simulink model "topology_2"  (R2024b)
settings: Solver=VariableStepAuto  StartTime=0.0  StopTime=1  RelTol=1e-3
undefined symbols (not defined in the file): C, L, par
libraries: spsSeriesRLCBranchLib x4, spsCurrentMeasurementLib x2, spsMosfetLib x2, spsVoltageMeasurementLib x2, spsDCVoltageSourceLib x1, spspowerguiLib x1
settings Model: Creator=marco  LastModifiedBy=marco

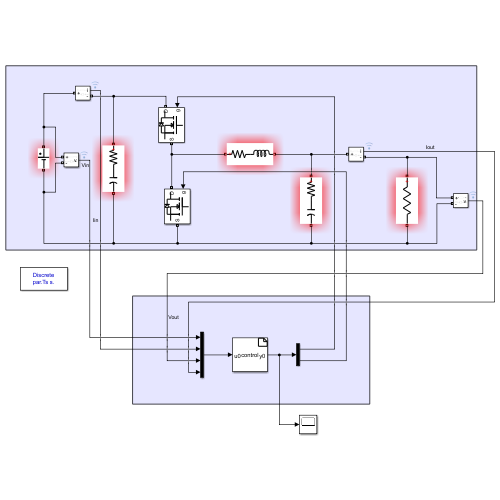
[thumbnail: Simulink's stored preview of the top-level diagram]
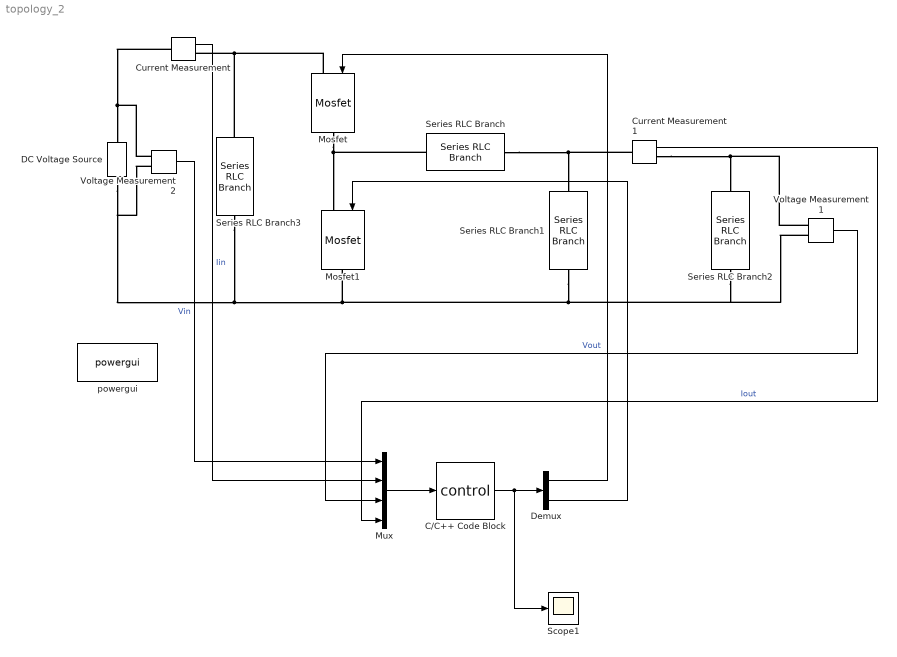
== system topology_2 ==
  C/C++ Code Block : S-Function  FunctionName=control  SFunctionModules=control_wrapper.c  SFunctionDeploymentMode=off  EnableBusSupport=off  mask(S-Function Builder){}
      mask help: Simulink:masks:SFunctionBuilder_MD
      mask init:
      | val = [[.9  0.75 0.75 1 1 .9 .9 1]',[1 1 0.75 0.75 .9 .9 1 .9]'];try , sys = get_param(gcb,'SfunBuilderFcnName');if isempty(sys), sys = get_param(gcb,'FunctionName'); end,catch, sys = get_param(gcb,'FunctionName'); end
      settings: CopyFcn=set_param(gcbh,'LinkStatus','none')  OpenFcn=sfunctionwizard(gcbh)
      mask Display:
      | plot(val(:,1),val(:,2))
      | disp(sys)
      | port_label('input',1,sprintf('%s', 'u0'),'interpreter','tex')
      | port_label('output',1,sprintf('%s', 'y0'),'interpreter','tex')
  Current Measurement : spsCurrentMeasurementLib/Current Measurement  PhasorSimulation=off  OutputType=Complex  PSBequivalent=0
  Current Measurement1 : spsCurrentMeasurementLib/Current Measurement  PhasorSimulation=off  OutputType=Complex  PSBequivalent=0
  DC Voltage Source : spsDCVoltageSourceLib/DC Voltage Source  Amplitude=par.V_source  Measurements=None
  Demux : Demux  Outputs=2
  Mosfet : spsMosfetLib/Mosfet  Ron=0.1  Lon=0  Rd=0.01  Vfd=0  IC=0  Rs=1e5  Cs=inf  Measurements=off
  Mosfet1 : spsMosfetLib/Mosfet  Ron=0.1  Lon=0  Rd=0.01  Vfd=0  IC=0  Rs=1e5  Cs=inf  Measurements=off
  Mux : Mux
  Scope1 : Scope
  Series RLC Branch : spsSeriesRLCBranchLib/Series RLC Branch  LConnTagsString=__new0  RConnTagsString=__new0  BranchType=RL  Resistance=par.R_L  Inductance=par.L  SetiL0=off  InitialCurrent=0  Capacitance=1e-6  Setx0=off  InitialVoltage=0  Measurements=None
  Series RLC Branch1 : spsSeriesRLCBranchLib/Series RLC Branch  LConnTagsString=__new0  RConnTagsString=__new0  BranchType=RC  Resistance=par.R_C  Inductance=L  SetiL0=off  InitialCurrent=0  Capacitance=par.C  Setx0=off  InitialVoltage=0  Measurements=None
  Series RLC Branch2 : spsSeriesRLCBranchLib/Series RLC Branch  LConnTagsString=__new0  RConnTagsString=__new0  BranchType=R  Resistance=par.R_load  Inductance=L  SetiL0=off  InitialCurrent=0  Capacitance=C  Setx0=off  InitialVoltage=0  Measurements=None
  Series RLC Branch3 : spsSeriesRLCBranchLib/Series RLC Branch  LConnTagsString=__new0  RConnTagsString=__new0  BranchType=RC  Resistance=par.R_C  Inductance=L  SetiL0=off  InitialCurrent=0  Capacitance=par.C  Setx0=off  InitialVoltage=0  Measurements=None
  Voltage Measurement1 : spsVoltageMeasurementLib/Voltage Measurement  PhasorSimulation=off  OutputType=Complex  PSBequivalent=0
  Voltage Measurement2 : spsVoltageMeasurementLib/Voltage Measurement  PhasorSimulation=off  OutputType=Complex  PSBequivalent=0
  powergui : spspowerguiLib/powergui  Priority=1  SimulationMode=Discrete  SampleTime=par.Ts  frequency=60  Iterations=50  frequencyindice=0  Pbase=100e6  ErrMax=1e-4  UnitsV=kV  UnitsW=MW  buscounter=0  FunctionMessages=off  echomessages=off  EnableUseOfTLC=off  CurrentSourceSwitches=off  DisableSnubberDevices=off  DisableRonSwitches=off  DisableVfSwitches=off  DisplayEquations=off  AutomaticDiscreteSolvers=off  SolverType=Tustin/Backward Euler (TBE)  Interpol=off  ExternalGateDelay=off  methode=off  Ts=100  x0status=blocks  SPID=on  SwTol=0  HookPort=off  NonlinearTolerance=1e-4  nMaxIteration=100  ContinueOnMaxIteration=off  RestoreLinks=warning  ResistiveCurrentMeasurement=off  Frange=[0:2:500]  Ylog=off  Xlog=on  ShowGrid=off  save=off  variable=ZData  structure=0  ZoomFFT=off  StartTime=0.0  cycles=1  DisplayStyle=1  fundamental=60  FreqAxis=off  MaxFrequency=1000  frequencyindicesteady=1  RmsSteady=1  display=off
  wires:
  C/C++ Code Block/1 -> Scope1/1, Demux/1
  Demux/1 -> Mosfet/1
  Demux/2 -> Mosfet1/1
  Voltage Measurement2/1 -> Mux/1  "Vin"
  Current Measurement/1 -> Mux/2  "Iin"
  Voltage Measurement1/1 -> Mux/3  "Vout"
  Current Measurement1/1 -> Mux/4  "Iout"
  Mux/1 -> C/C++ Code Block/1
  connections:
  Series RLC Branch1/RConn1 -- Series RLC Branch2/RConn1 -- Voltage Measurement1/LConn2 -- Voltage Measurement2/LConn2 -- DC Voltage Source/LConn1 -- Series RLC Branch3/RConn1 -- Mosfet1/RConn1
  Mosfet/RConn1 -- Series RLC Branch/LConn1 -- Mosfet1/LConn1
  Series RLC Branch/RConn1 -- Current Measurement1/LConn1 -- Series RLC Branch1/LConn1
  Mosfet/LConn1 -- Current Measurement/RConn1 -- Series RLC Branch3/LConn1
  Current Measurement/LConn1 -- Voltage Measurement2/LConn1 -- DC Voltage Source/RConn1
  Voltage Measurement1/LConn1 -- Current Measurement1/RConn1 -- Series RLC Branch2/LConn1
